simulink model "Top_Level"  (Simulink 7.5)
settings: Solver=ode45  StartTime=0.0  StopTime=inf  RelTol=1e-3
undefined symbols (not defined in the file): dfilt, DiscIntNeverNeededParam, fspecial, gray, Horn, imresize, Low, Rec, Schunck, SDTV
libraries: simulink x13, dspobslib x10, dspsigops x4, vipgeotforms x4, viptextngfix x4, vipsnks x3, dspmtrx3 x2, vipanalysis x2, vipconversions x1, dsparch4 x1, dspswit3 x1, vipsrcs x1
(part 1 of 2)
settings Model: Creator=roczit00  LastModifiedBy=Anonymos
settings DebuggingCC: AlgebraicLoopMsg=none  SolverPrmCheckMsg=none  UnconnectedInputMsg=none  UnconnectedOutputMsg=none  UnconnectedLineMsg=none  StrictBusMsg=Warning

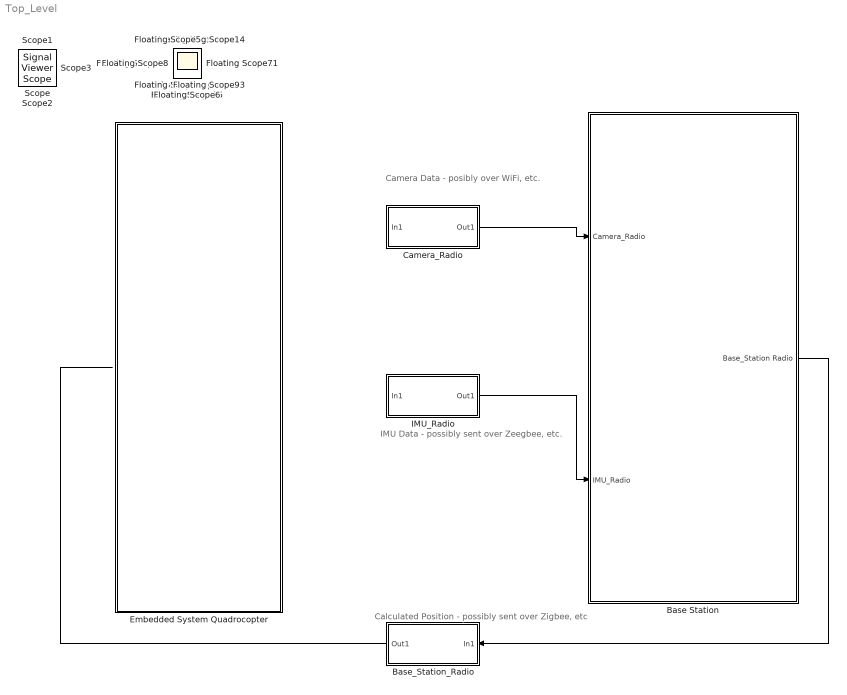
== system Top_Level ==
  note: IMU Data - possibly sent over Zeegbee, etc.
  note: Calculated Position - possibly sent over Zigbee, etc
  note: Camera Data - posibly over WiFi, etc.
  Base Station : Subsystem
  Base_Station_Radio : Subsystem
  Camera_Radio : Subsystem
  Embedded System Quadrocopter : Subsystem
  IMU_Radio : Subsystem
  Floating Scope{,1..15} (16 alike) : Scope
      Floating Scope settings: Floating=on  YMin=-40  YMax=90
      Floating Scope1 settings: Floating=on
      Floating Scope10 settings: Floating=on  SaveName=ScopeData12
      Floating Scope11 settings: Floating=on  SaveName=ScopeData13
      Floating Scope12 settings: Floating=on  YMin=-2500  YMax=27500  SaveName=ScopeData14
      Floating Scope13 settings: Floating=on  SaveName=ScopeData16
      Floating Scope14 settings: Floating=on  SaveName=ScopeData17
      Floating Scope15 settings: Floating=on  YMin=-2.5  YMax=27.5  SaveName=ScopeData18
      Floating Scope2 settings: Floating=on  YMin=-6000  YMax=2500  SaveName=ScopeData2
      Floating Scope3 settings: Floating=on  SaveName=ScopeData3
      Floating Scope4 settings: Floating=on  SaveName=ScopeData4
      Floating Scope5 settings: Floating=on  YMin=-0.7  YMax=0.8  SaveName=ScopeData5
      Floating Scope6 settings: Floating=on  YMin=-1  YMax=1  SaveName=ScopeData6
      Floating Scope7 settings: Floating=on  YMin=-15  YMax=10  SaveName=ScopeData7
      Floating Scope8 settings: Floating=on  YMax=45  SaveName=ScopeData10
      Floating Scope9 settings: Floating=on  YMin=-2  YMax=6.5  SaveName=ScopeData11
  Scope{,1..3} (4 alike) : SignalViewerScope  IOType=viewer  RefreshTime=0.035000
      Scope settings: YMin=-0.01  YMax=0.1
      Scope2 settings: SaveName=ScopeData2
      Scope3 settings: SaveName=ScopeData3
  wires:
  ? -> Camera_Radio/1(In1)
  Base Station/1(Base_Station Radio) -> Base_Station_Radio/1(In1)
  Base_Station_Radio/1(Out1) -> ?
  ? -> IMU_Radio/1(In1)
  IMU_Radio/1(Out1) -> Base Station/2(IMU_Radio)
  Camera_Radio/1(Out1) -> Base Station/1(Camera_Radio)

== system Top_Level/Base Station ==
  Camera_Radio : Inport
  IMU_Radio : Inport  Port=2
  Allow Image Processing : dspobslib/DSP Constant  SystemSampleTime=-1  Value=1  SampleMode=Discrete  discreteOutput=Sample-based  continuousOutput=Sample-based  sampTime=inf  framePeriod=2  dataType=boolean  isSigned=on  wordLen=16  udDataType=sfix(16)  fracBitsMode=Best precision  numFracBits=15  InterpretAs1D=-inf  Ts=-inf  FramebasedOutput=-inf
  Disable Image Processing : dspobslib/DSP Constant  SystemSampleTime=-1  Value=0  SampleMode=Discrete  discreteOutput=Sample-based  continuousOutput=Sample-based  sampTime=inf  framePeriod=2  dataType=boolean  isSigned=on  wordLen=16  udDataType=sfix(16)  fracBitsMode=Best precision  numFracBits=15  InterpretAs1D=-inf  Ts=-inf  FramebasedOutput=-inf
  Image Processing : Subsystem
  Selector1 : Selector  InputPortWidth=19  IndexOptions=Index vector (dialog)  Indices=[7 8 12]  OutputSizes=1
  Switch1 : simulink/Signal Routing/Manual Switch  SystemSampleTime=-1  sw=1  action=0  varsize=off
  Base_Station Radio : Outport
  wires:
  Camera_Radio/1 -> Selector1/1, Image Processing/1("x, y, vel_psi")
  Selector1/1 -> Base_Station Radio/1
  Allow Image Processing/1 -> Switch1/1
  Disable Image Processing/1 -> Switch1/2
  Switch1/1 -> Image Processing/Enable

== system Top_Level/Base_Station_Radio ==
  In1 : Inport
  Out1 : Outport
  wires:
  In1/1 -> Out1/1

== system Top_Level/Camera_Radio ==
  In1 : Inport
  Demux : Demux  Outputs=3
  Mux : Mux  Inputs=3
  Out1 : Outport
  wires:
  In1/1 -> Demux/1
  Demux/2 -> Mux/2
  Demux/3 -> Mux/3
  Demux/1 -> Mux/1
  Mux/1 -> Out1/1

== system Top_Level/Embedded System Quadrocopter ==

== system Top_Level/IMU_Radio ==
  In1 : Inport
  Out1 : Outport
  wires:
  In1/1 -> Out1/1

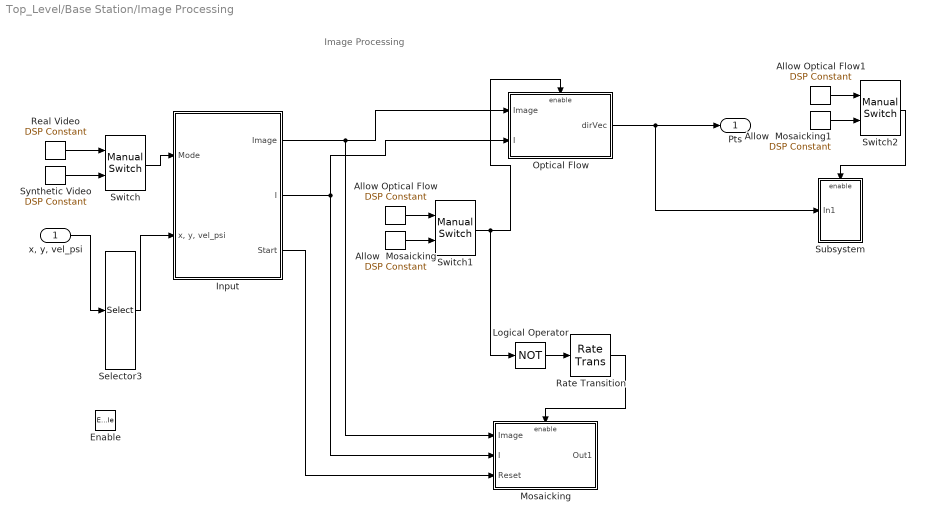
== system Top_Level/Base Station/Image Processing ==
  note: Image Processing
  "x, y, vel_psi" : Inport
  Enable : EnablePort  PropagateVarSize=During execution
  Allow  Mosaicking : dspobslib/DSP Constant  SystemSampleTime=-1  Value=0  SampleMode=Discrete  discreteOutput=Sample-based  continuousOutput=Sample-based  sampTime=inf  framePeriod=2  dataType=boolean  isSigned=on  wordLen=16  udDataType=sfix(16)  fracBitsMode=Best precision  numFracBits=15  InterpretAs1D=-inf  Ts=-inf  FramebasedOutput=-inf
  Allow  Mosaicking1 : dspobslib/DSP Constant  SystemSampleTime=-1  Value=0  SampleMode=Discrete  discreteOutput=Sample-based  continuousOutput=Sample-based  sampTime=inf  framePeriod=2  dataType=boolean  isSigned=on  wordLen=16  udDataType=sfix(16)  fracBitsMode=Best precision  numFracBits=15  InterpretAs1D=-inf  Ts=-inf  FramebasedOutput=-inf
  Allow Optical Flow : dspobslib/DSP Constant  SystemSampleTime=-1  Value=1  SampleMode=Discrete  discreteOutput=Sample-based  continuousOutput=Sample-based  sampTime=inf  framePeriod=2  dataType=boolean  isSigned=on  wordLen=16  udDataType=sfix(16)  fracBitsMode=Best precision  numFracBits=15  InterpretAs1D=-inf  Ts=-inf  FramebasedOutput=-inf
  Allow Optical Flow1 : dspobslib/DSP Constant  SystemSampleTime=-1  Value=1  SampleMode=Discrete  discreteOutput=Sample-based  continuousOutput=Sample-based  sampTime=inf  framePeriod=2  dataType=boolean  isSigned=on  wordLen=16  udDataType=sfix(16)  fracBitsMode=Best precision  numFracBits=15  InterpretAs1D=-inf  Ts=-inf  FramebasedOutput=-inf
  Input : Subsystem
  Logical Operator : Logic  Operator=NOT  AllPortsSameDT=off  OutDataTypeMode=boolean  OutDataTypeStr=boolean
  Mosaicking : Subsystem
  Optical Flow : Subsystem
  Rate Transition : RateTransition  OutPortSampleTimeOpt=Inherit
  Real Video : dspobslib/DSP Constant  SystemSampleTime=-1  Value=0  SampleMode=Discrete  discreteOutput=Sample-based  continuousOutput=Sample-based  sampTime=inf  framePeriod=2  dataType=boolean  isSigned=on  wordLen=16  udDataType=sfix(16)  fracBitsMode=Best precision  numFracBits=15  InterpretAs1D=-inf  Ts=-inf  FramebasedOutput=-inf
  Selector3 : Selector  InputPortWidth=19  IndexOptions=Index vector (dialog)  Indices=[1 2 6]  OutputSizes=1
  Subsystem : Subsystem
  Switch : simulink/Signal Routing/Manual Switch  SystemSampleTime=-1  sw=0  action=0  varsize=off
  Switch1 : simulink/Signal Routing/Manual Switch  SystemSampleTime=-1  sw=1  action=0  varsize=off
  Switch2 : simulink/Signal Routing/Manual Switch  SystemSampleTime=-1  sw=1  action=0  varsize=off
  Synthetic Video : dspobslib/DSP Constant  SystemSampleTime=-1  Value=1  SampleMode=Discrete  discreteOutput=Sample-based  continuousOutput=Sample-based  sampTime=inf  framePeriod=2  dataType=boolean  isSigned=on  wordLen=16  udDataType=sfix(16)  fracBitsMode=Best precision  numFracBits=15  InterpretAs1D=-inf  Ts=-inf  FramebasedOutput=-inf
  Pts : Outport  OutDataType=fixdt(1, 16)  OutScaling=2^0
  wires:
  Real Video/1 -> Switch/1
  Synthetic Video/1 -> Switch/2
  Switch/1 -> Input/1(Mode)
  "x, y, vel_psi"/1 -> Selector3/1
  Optical Flow/1(dirVec) -> Pts/1, Subsystem/1(In1)
  Input/1(Image) -> Mosaicking/1(Image), Optical Flow/1(Image)
  Input/2(I) -> Mosaicking/2(I), Optical Flow/2(I)
  Switch1/1 -> Optical Flow/Enable, Logical Operator/1
  Logical Operator/1 -> Rate Transition/1
  Rate Transition/1 -> Mosaicking/Enable
  Input/3(Start) -> Mosaicking/3(Reset)
  Allow Optical Flow/1 -> Switch1/1
  Allow  Mosaicking/1 -> Switch1/2
  Selector3/1 -> Input/2("x, y, vel_psi")
  Allow Optical Flow1/1 -> Switch2/1
  Allow  Mosaicking1/1 -> Switch2/2
  Switch2/1 -> Subsystem/Enable

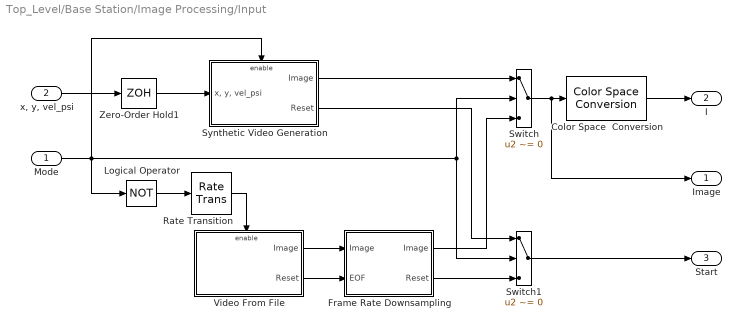
== system Top_Level/Base Station/Image Processing/Input ==
  Mode : Inport  OutDataType=sfix(16)  OutScaling=2^0
  "x, y, vel_psi" : Inport  Port=2  OutDataType=sfix(16)  OutScaling=2^0
  Color Space  Conversion : vipconversions/Color Space  Conversion  conversion=Obsolete  conversionActive=R'G'B' to intensity  wp_str=D65  rec=Rec. 601 (SDTV)  sys=1125/60/2:1  imagePorts=One multidimensional signal
  Frame Rate Downsampling : Subsystem  mask(Select Video Frames){frameRate=1}
      mask prompts: frameRate "N:"
      mask help: Downsample the video sequence by processing every Nth frame.
      mask init:
      | switch frameRate
      |     case 1,
      |         icon = sprintf('Select\nAll Frames');
      |     case 2,
      |         icon = sprintf('Select Every\n2nd Frame');
      |     case 3,
      |         icon = sprintf('Select Every\n3rd Frame');
      |     otherwise,
      |         icon = sprintf('Select Every\n%dth Frame',frameRate);
      | end
      mask Display: disp(icon);
  Logical Operator : Logic  Operator=NOT  AllPortsSameDT=off  OutDataTypeMode=boolean  OutDataTypeStr=boolean
  Rate Transition : RateTransition  OutPortSampleTimeOpt=Inherit
  Switch : Switch  Criteria=u2 ~= 0  OutDataType=sfix(16)  OutScaling=2^0
  Switch1 : Switch  Criteria=u2 ~= 0  OutDataType=sfix(16)  OutScaling=2^0
  Synthetic Video Generation : Subsystem  mask(Synthetic Video Generation){dimen=[288 352], origin=[509 765], velocity=[5 10], varVelocity=[8 5], varCorner=[10 10], rotation=1, varRotation=0.2}
      mask prompts: dimen "Size of the synthetic image:"; origin "Initial image center:"; varVelocity "Variance of velocity:"; varCorner "Variance of corner location:"; rotation "Rotation speed (in degrees):"; varRotation "Variation of rotation (in degrees):"
      mask help: Generates a synthetic video.
  Video From File : Subsystem
  Zero-Order Hold1 : ZeroOrderHold  SampleTime=0.01
  Image : Outport
  I : Outport  Port=2
  Start : Outport  Port=3
  wires:
  Switch1/1 -> Start/1
  Switch/1 -> Image/1, Color Space  Conversion/1
  Logical Operator/1 -> Rate Transition/1
  Rate Transition/1 -> Video From File/Enable
  Synthetic Video Generation/2(Reset) -> Switch1/1
  Synthetic Video Generation/1(Image) -> Switch/1
  Mode/1 -> Logical Operator/1, Switch1/2, Switch/2, Synthetic Video Generation/Enable
  Video From File/1(Image) -> Frame Rate Downsampling/1(Image)
  Video From File/2(Reset) -> Frame Rate Downsampling/2(EOF)
  Frame Rate Downsampling/1("Image ") -> Switch/3
  Frame Rate Downsampling/2(Reset) -> Switch1/3
  "x, y, vel_psi"/1 -> Zero-Order Hold1/1
  Zero-Order Hold1/1 -> Synthetic Video Generation/1("x, y, vel_psi")
  Color Space  Conversion/1 -> I/1

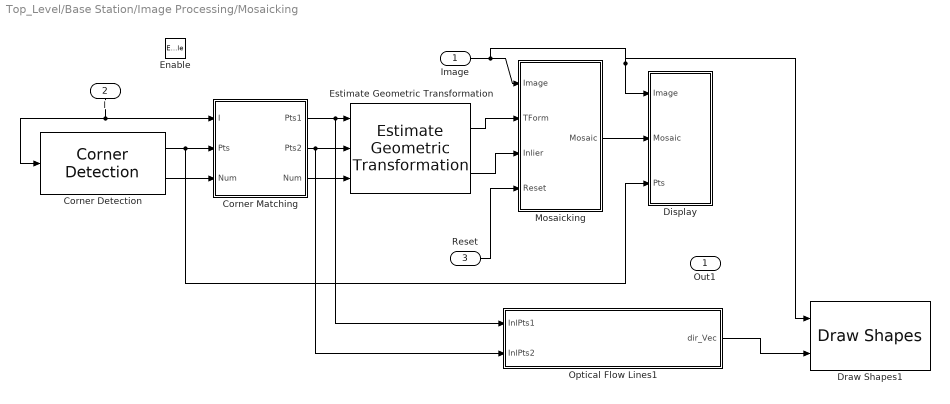
== system Top_Level/Base Station/Image Processing/Mosaicking ==
  Image : Inport
  I : Inport  Port=2
  Reset : Inport  Port=3
  Enable : EnablePort  PropagateVarSize=During execution
  Corner Detection : vipanalysis/Corner Detection  DialogController=vipDDGCreate  DialogControllerArgs=DataTag5  SystemSampleTime=-1  method=Local intensity comparison (Rosen & Drummond)  factor=0.04  filter=fspecial('gaussian', [1 5], 1.5)  thrInten=0.1  thrAngle=157.5  output=Corner location  outputInUse=Corner location  maxNum=75  thrMetric=0.001  neighborSize=[21 21]  isOutVarDim=on  accumMode=Binary point scaling  accumWordLength=32  accumFracLength=0  prodOutputMode=Binary point scaling  prodOutputWordLength=32  prodOutputFracLength=0  memoryMode=Binary point scaling  memoryWordLength=32  memoryFracLength=0  firstCoeffMode=Specify word length  firstCoeffWordLength=16  firstCoeffFracLength=16  roundingMode=Floor  overflowMode=off
  Corner Matching : Subsystem  mask(Corner Matching){winLen=9, maxNum=75, threshold=81}
      mask prompts: winLen "Block size used in corner matching:"; maxNum "Maximum number of points:"; threshold "Maximum feature difference for matching points:"
      mask help: Find out matching corners in the current and previous video frames.
  Display : Subsystem
  Draw Shapes1 : viptextngfix/Draw Shapes  DialogController=vipDDGCreate  DialogControllerArgs=DataTag13  shape=Lines  fill=off  fillClrSource=Specify via dialog  display=User-specified value  intensity=200  color=[255 255 0]  opacity=0.6  viewport=Entire image  antialiasing=off  inType=Obsolete  imagePorts=One multidimensional signal  prodOutputMode=Binary point scaling  prodOutputWordLength=32  prodOutputFracLength=14  memoryMode=Specify word length  memoryWordLength=16  memoryFracLength=15  roundingMode=Floor  overflowMode=off
  Estimate Geometric Transformation : vipgeotforms/Estimate Geometric Transformation  DialogController=vipDDGCreate  DialogControllerArgs=DataTag14  tformType=Projective  isRandomSampling=on  algMethod=Random Sample Consensus (RANSAC)  numMethod=Desired confidence  isStopSampling=on  percentStop=75  distanceAlg=1  distanceGeo=1.5  sampleNum=500  maxSampleNum=500  desiredConfidence=99  isRefineTForm=on  isOutputInlier=on  outDT4IntInput=Obsolete10a  outDT4IntInputActive=Single  isVarSizeAllowed=off  isReleaseMode=on
  Mosaicking : Subsystem  mask(Mosaicking){sizePano=[400 670], orginPano=[60 5]}
      mask prompts: sizePano "Size of the mosaic image:"; orginPano "Initial image placement (top-left image boundary):"
      mask help: Overlay video frames to create mosaic image.
  Optical Flow Lines1 : Stateflow chart  TreatAsAtomicUnit=on
  Out1 : Outport  OutDataType=fixdt(1, 16)  OutScaling=2^0
  wires:
  Corner Detection/1 -> Corner Matching/2(Pts), Display/3(Pts)
  Corner Detection/2 -> Corner Matching/3(Num)
  Mosaicking/1(Mosaic) -> Display/2(Mosaic)
  Corner Matching/1(Pts1) -> Estimate Geometric Transformation/1, Optical Flow Lines1/1(InlPts1)
  Corner Matching/2(Pts2) -> Estimate Geometric Transformation/2, Optical Flow Lines1/2(InlPts2)
  Corner Matching/3("Num ") -> Estimate Geometric Transformation/3
  Estimate Geometric Transformation/2 -> Mosaicking/3(Inlier)
  Estimate Geometric Transformation/1 -> Mosaicking/2(TForm)
  Image/1 -> Mosaicking/1(Image), Display/1(Image), Draw Shapes1/1
  I/1 -> Corner Detection/1, Corner Matching/1(I)
  Reset/1 -> Mosaicking/4(Reset)
  Optical Flow Lines1/1(dir_Vec) -> Draw Shapes1/2

== system Top_Level/Base Station/Image Processing/Optical Flow ==
  note: Optical Flow Movement Detection
  Image : Inport
  I : Inport  Port=2
  Enable : EnablePort  PropagateVarSize=During execution
  Allow draw lines : dspobslib/DSP Constant  SystemSampleTime=-1  Value=1  SampleMode=Discrete  discreteOutput=Sample-based  continuousOutput=Sample-based  sampTime=inf  framePeriod=2  dataType=boolean  isSigned=on  wordLen=16  udDataType=sfix(16)  fracBitsMode=Best precision  numFracBits=15  InterpretAs1D=-inf  Ts=-inf  FramebasedOutput=-inf
  Disable draw lines : dspobslib/DSP Constant  SystemSampleTime=-1  Value=0  SampleMode=Discrete  discreteOutput=Sample-based  continuousOutput=Sample-based  sampTime=inf  framePeriod=2  dataType=boolean  isSigned=on  wordLen=16  udDataType=sfix(16)  fracBitsMode=Best precision  numFracBits=15  InterpretAs1D=-inf  Ts=-inf  FramebasedOutput=-inf
  Optical Flow Lines1 : Subsystem  mask(Optical Flow Lines){scaleFactor=0.0008}
      mask prompts: scaleFactor "Motion vector gain:"
      mask help: Generates the coordinate points of optical flow lines.
      mask Help: Generates the coordinate points of optical flow lines. Look under its mask to see the implementation details.
  Optical Flow1 : vipanalysis/Optical Flow  DialogController=vipDDGCreate  DialogControllerArgs=DataTag17  SystemSampleTime=-1  method=Horn-Schunck  gradMethod=Derivative of Gaussian  which2img=Current frame and N-th frame back  N=1  outVelForm=Horizontal and vertical components in complex form  lambda=0.01  stop_criteria=When maximum number of iterations is reached  maxAllowAbsDiff=eps  maxIter=10  numInports=3  sigmaS=1.5  sigmaW=1  eigTh=0.0039  discardNormalFlow=off  outputCurrentImage=on  prodOutputMode=Binary point scaling  prodOutputWordLength=32  prodOutputFracLength=20  outputMode=Binary point scaling  outputWordLength=32  outputFracLength=20  roundingMode=Nearest  overflowMode=on
  Subsystem : Subsystem
  Switch2 : simulink/Signal Routing/Manual Switch  SystemSampleTime=-1  sw=1  action=0  varsize=off
  dirVec : Outport  OutDataType=fixdt(1, 16)  OutScaling=2^0
  wires:
  Optical Flow1/1 -> Optical Flow Lines1/1(vel.Values)
  Optical Flow Lines1/1(vel.Lines) -> Subsystem/2(In2)
  Image/1 -> Subsystem/1(In1)
  I/1 -> Optical Flow1/1
  Optical Flow Lines1/2(dirVec) -> dirVec/1
  Allow draw lines/1 -> Switch2/1
  Disable draw lines/1 -> Switch2/2
  Switch2/1 -> Subsystem/Enable

== system Top_Level/Base Station/Image Processing/Subsystem ==
  In1 : Inport
  Enable : EnablePort  PropagateVarSize=During execution
  Demux : Demux  Outputs=2
  Discrete-Time Integrator : DiscreteIntegrator  SampleTime=-1  OutDataType=fixdt(1, 16)  OutScaling=2^0  ICPrevOutput=DiscIntNeverNeededParam  ICPrevScaledInput=DiscIntNeverNeededParam
  Gain1 : Gain  Gain=-1  ParameterDataType=fixdt(1, 16)  ParameterScaling=2^0  OutDataType=fixdt(1, 16)  OutScaling=2^0
  XY Pos. Est : simulink/Sinks/XY Graph  SystemSampleTime=-1  xmin=-10  xmax=10  ymin=-10  ymax=10  st=-1
  wires:
  Discrete-Time Integrator/1 -> Demux/1
  Demux/1 -> XY Pos. Est/1
  Demux/2 -> Gain1/1
  Gain1/1 -> XY Pos. Est/2
  In1/1 -> Discrete-Time Integrator/1

== system Top_Level/Base Station/Image Processing/Input/Frame Rate Downsampling ==
  Image : Inport  OutDataType=sfix(16)  OutScaling=2^0
  EOF : Inport  Port=2  OutDataType=sfix(16)  OutScaling=2^0
  Compare To Zero : simulink/Logic and Bit Operations/Compare To Zero  SystemSampleTime=-1  relop=>  LogicOutDataTypeMode=boolean  ZeroCross=off
  Data Type Conversion : DataTypeConversion  OutDataTypeMode=single  OutDataType=sfix(16)  OutScaling=2^0  OutDataTypeStr=single
  Digital Filter : dsparch4/Digital Filter  DialogController=dspdialog.DigitalFilter  DialogControllerArgs=DataTag0  TypePopup=FIR (all zeros)  IIRFiltStruct=Direct form II transposed  AllPoleFiltStruct=Direct form  FIRFiltStruct=Direct form  CoeffSource=Specify via dialog  NumCoeffs=ones(1, frameRate)  DenCoeffs=[1 0.1]  BiQuadCoeffs=[1 0.3 0.4 1 0.1 0.2]  LatticeCoeffs=[0.2 0.4]  denIgnore=on  FiltPerSampPopup=One filter per frame  IC=0  ICnum=0  ICden=0  roundingMode=Floor  overflowMode=off  ScaleValues=1  scaleValueFracLength=14  stageInFracLength=15  stageOutFracLength=15  FilterSource=Specify via dialog  dfiltObjectName=dfilt.dffir([1 2 1])
  Downsample : dspsigops/Downsample  N=frameRate  phase=0  ic=0  smode=Allow multirate  fmode=Maintain input frame size
  Downsample3 : dspsigops/Downsample  N=frameRate  phase=0  ic=0  smode=Allow multirate  fmode=Maintain input frame size
  Unit Delay : UnitDelay  X0=1  SampleTime=-1
  "Image " : Outport  OutDataType=sfix(16)  OutScaling=2^0
  Reset : Outport  Port=2
  wires:
  Digital Filter/1 -> Compare To Zero/1
  Data Type Conversion/1 -> Digital Filter/1
  Compare To Zero/1 -> Unit Delay/1
  Downsample3/1 -> Reset/1
  EOF/1 -> Data Type Conversion/1
  Unit Delay/1 -> Downsample3/1
  Image/1 -> Downsample/1
  Downsample/1 -> "Image "/1

== system Top_Level/Base Station/Image Processing/Input/Synthetic Video Generation ==
  "x, y, vel_psi" : Inport  OutDataType=sfix(16)  OutScaling=2^0
  Enable : EnablePort  PropagateVarSize=During execution
  N-Sample Enable : dspswit3/N-Sample Enable  N=1  ActiveLevel=Low (0)  reset=off  TriggerType=Rising edge  Ts=-1  DataType=Logical
  Read Image : Subsystem
      settings: AttributesFormatString=Load image only at the beginning of simulation
  Synthesize Video : Subsystem  mask{dimen=dimen, origin=origin, velocity=velocity, varVelocity=varVelocity, varCorner=varCorner, rotation=rotation, varRotation=varRotation}
      mask prompts: dimen "Size of the synthetic image:"; origin "Initial image center:"; varVelocity "Variance of velocity:"; varCorner "Variance of corner location:"; rotation "Rotation speed:"; varRotation "Variation of rotation:"
  Image : Outport
  Reset : Outport  Port=2  InitialOutput=1
  wires:
  Read Image/2(Size) -> Synthesize Video/2(Size)
  Read Image/1(Image) -> Synthesize Video/1("Image ")
  N-Sample Enable/1 -> Read Image/Enable
  Synthesize Video/2(Reset) -> Reset/1
  Synthesize Video/1(Image) -> Image/1
  "x, y, vel_psi"/1 -> Synthesize Video/3("x, y, vel_psi")

== system Top_Level/Base Station/Image Processing/Input/Video From File ==
  Enable : EnablePort  PropagateVarSize=During execution
  From Multimedia File : dspsrcs4/From Multimedia File  DialogController=dspDDGCreate  DialogControllerArgs=DataTag4  inputFilename=D:\_HSE\_ARBEIT\eclipse-cpp-galileo-SR1-win32\Workspace2\MASTER_THESIS_PRJ\scratch\Ground_Videos\grey_amorphic_flow_tiles_variable_light.avi  loop=on  numPlays=inf  outputStreams=Video only  videoDataType=single  audioDataType=int16  inheritSampleTime=on  userDefinedSampleTime=1/30  noAudioOutput=off  isIntensityVideo=off  fourcc=RGB  colorVideoFormat=One multidimensional signal  outputEOF=on  dataOrg=Column-major  audioFrameSize=1024  computeAudioFrameSize=off
  Image : Outport
  Reset : Outport  Port=2
  wires:
  From Multimedia File/1 -> Image/1
  From Multimedia File/2 -> Reset/1

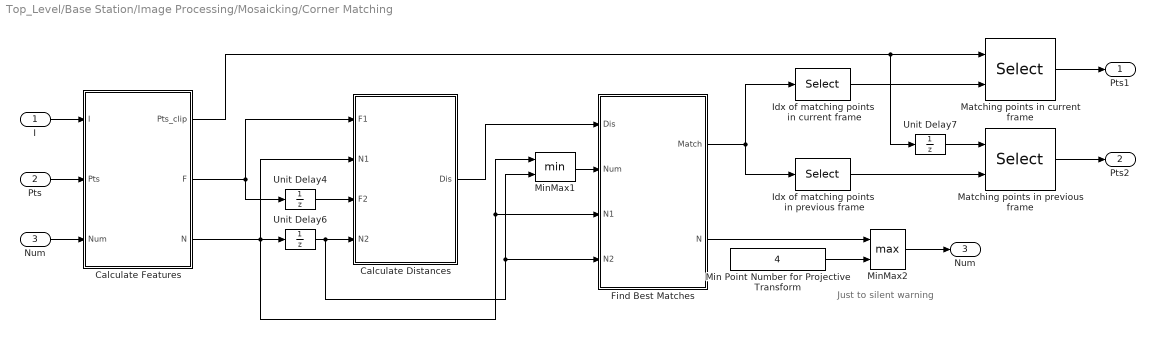
== system Top_Level/Base Station/Image Processing/Mosaicking/Corner Matching ==
  note: Just to
      | silent warning
  I : Inport  OutDataType=sfix(16)  OutScaling=2^0
  Pts : Inport  Port=2  OutDataType=sfix(16)  OutScaling=2^0
  Num : Inport  Port=3  OutDataType=sfix(16)  OutScaling=2^0
  Calculate Distances : Subsystem  TreatAsAtomicUnit=on  mask{maxNum=maxNum}
      mask prompts: maxNum "Maximum data number:"
      settings: AttributesFormatString=between features.
  Calculate Features : Subsystem  TreatAsAtomicUnit=on  mask{winLen=winLen, maxNum=maxNum}
      mask prompts: winLen "Neighborhood size:"; maxNum "Maximum number of features:"
  Find Best Matches : Subsystem  TreatAsAtomicUnit=on  mask{maxNum=maxNum, threshold=threshold}
      mask prompts: maxNum "Maximum data number:"
      settings: AttributesFormatString=between the features\nin the current and previous frames
  Idx of matching points  in current frame : Selector  NumberOfDimensions=2  IndexMode=Zero-based  InputPortWidth=2  IndexOptions=Index vector (dialog),Select all  Indices=0,1  OutputSizes=1,1
  Idx of matching points  in previous frame : Selector  NumberOfDimensions=2  IndexMode=Zero-based  InputPortWidth=2  IndexOptions=Index vector (dialog),Select all  Indices=1,1  OutputSizes=1,1
  Matching points in current frame : Selector  NumberOfDimensions=2  IndexMode=Zero-based  InputPortWidth=2  IndexOptions=Select all,Index vector (port)  Indices=0,1  OutputSizes=1,1
  Matching points in previous frame : Selector  NumberOfDimensions=2  IndexMode=Zero-based  InputPortWidth=2  IndexOptions=Select all,Index vector (port)  Indices=0,1  OutputSizes=1,1
  Min Point Number for Projective Transform : Constant  Value=4  OutDataType=sfix(16)  OutScaling=2^0  OutDataTypeStr=Inherit: Inherit via back propagation
  MinMax1 : MinMax  Inputs=2  OutDataType=sfix(16)  OutScaling=2^0
  MinMax2 : MinMax  Function=max  Inputs=2  OutDataType=sfix(16)  OutScaling=2^0  OutDataTypeStr=Inherit: Inherit via back propagation
  Unit Delay4 : UnitDelay  SampleTime=-1
  Unit Delay6 : UnitDelay  SampleTime=-1
  Unit Delay7 : UnitDelay  SampleTime=-1
  Pts1 : Outport  OutDataType=sfix(16)  OutScaling=2^0
  Pts2 : Outport  Port=2  OutDataType=sfix(16)  OutScaling=2^0
  "Num " : Outport  Port=3  OutDataType=sfix(16)  OutScaling=2^0
  wires:
  Calculate Features/2(F) -> Calculate Distances/1(F1), Unit Delay4/1
  Calculate Features/3(N) -> Calculate Distances/2(N1), Unit Delay6/1, MinMax1/1, Find Best Matches/3(N1)
  Calculate Features/1(Pts_clip) -> Unit Delay7/1, Matching points in current frame/1
  Num/1 -> Calculate Features/3(Num)
  Unit Delay6/1 -> Calculate Distances/4(N2), MinMax1/2, Find Best Matches/4(N2)
  Unit Delay4/1 -> Calculate Distances/3(F2)
  Matching points in previous frame/1 -> Pts2/1
  Matching points in current frame/1 -> Pts1/1
  Unit Delay7/1 -> Matching points in previous frame/1
  Idx of matching points  in current frame/1 -> Matching points in current frame/2
  Idx of matching points  in previous frame/1 -> Matching points in previous frame/2
  Find Best Matches/1(Match) -> Idx of matching points  in previous frame/1, Idx of matching points  in current frame/1
  Calculate Distances/1(Dis) -> Find Best Matches/1(Dis)
  I/1 -> Calculate Features/1(I)
  Pts/1 -> Calculate Features/2(Pts)
  Min Point Number for Projective Transform/1 -> MinMax2/2
  Find Best Matches/2(N) -> MinMax2/1
  MinMax2/1 -> "Num "/1
  MinMax1/1 -> Find Best Matches/2(Num)

== system Top_Level/Base Station/Image Processing/Mosaicking/Display ==
  Image : Inport  OutDataType=sfix(16)  OutScaling=2^0
  Mosaic : Inport  Port=2  OutDataType=sfix(16)  OutScaling=2^0
  Pts : Inport  Port=3  OutDataType=sfix(16)  OutScaling=2^0
  Corners : vipsnks/Video Viewer  DialogControllerArgs=DataTag9  inputType=Obsolete7b  imagePorts=One multidimensional signal  useColorMap=off  colormapValue=gray(256)  specRange=off  minInputVal=0  maxInputVal=255  FigPos=[1 766 1276 659]  AxisZoom=on  trueSizedOnce=on  OpenAtMdlStart=on
  Draw Corners : viptextngfix/Draw Markers  DialogController=vipDDGCreate  DialogControllerArgs=DataTag10  shape=Circle  size=3  fill=off  fillClrSource=Specify via dialog  display=User-specified value  intensity=155  color=[1 0 0]  opacity=1  viewport=Entire image  antialiasing=off  inType=Obsolete  imagePorts=One multidimensional signal  prodOutputMode=Binary point scaling  prodOutputWordLength=32  prodOutputFracLength=14  memoryMode=Specify word length  memoryWordLength=16  memoryFracLength=15  roundingMode=Floor  overflowMode=off
  "Mosaic " : vipsnks/Video Viewer  DialogControllerArgs=DataTag12  inputType=Obsolete7b  imagePorts=One multidimensional signal  useColorMap=off  colormapValue=gray(256)  specRange=off  minInputVal=0  maxInputVal=255  FigPos=[12 653 673 423]  AxisZoom=on  trueSizedOnce=on  OpenAtMdlStart=on
  wires:
  Mosaic/1 -> "Mosaic "/1
  Image/1 -> Draw Corners/1
  Draw Corners/1 -> Corners/1
  Pts/1 -> Draw Corners/2

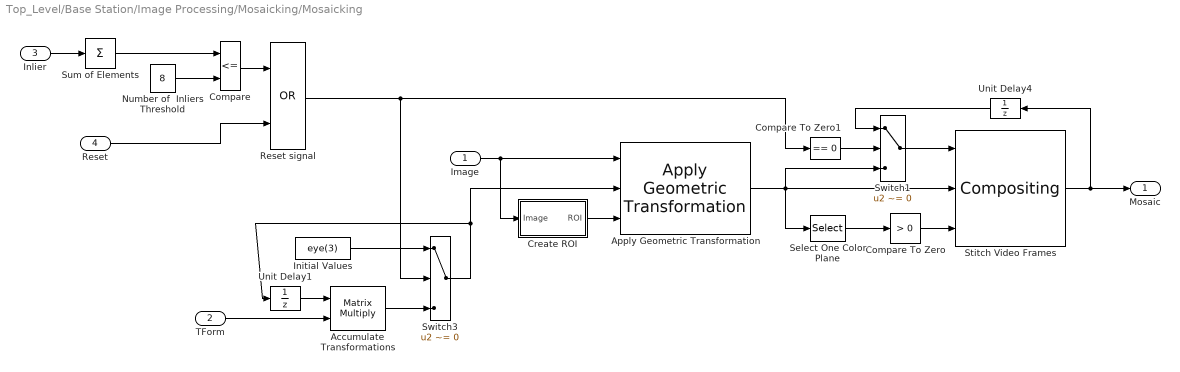
== system Top_Level/Base Station/Image Processing/Mosaicking/Mosaicking ==
  Image : Inport  OutDataType=sfix(16)  OutScaling=2^0
  TForm : Inport  Port=2  OutDataType=sfix(16)  OutScaling=2^0
  Inlier : Inport  Port=3  OutDataType=sfix(16)  OutScaling=2^0
  Reset : Inport  Port=4  OutDataType=sfix(16)  OutScaling=2^0
  Accumulate Transformations : Product  Multiplication=Matrix(*)  OutDataType=sfix(16)  OutScaling=2^0  RndMeth=Zero  InputSameDT=on
  Apply Geometric Transformation : vipgeotforms/Apply Geometric Transformation  DialogController=vipDDGCreate  DialogControllerArgs=DataTag15  tformSource=Input port  tformValue=[1 0 0; 0 1 0; 0 0 1]  approxProjectiveFlag=off  errorTolerance=1.0  roiMethod=Rectangle ROI  roiSource=Input port  roiBBox=[0 0 128 256]  roiVertice=[0 0 10 12 20 22]  inputClipFlag=off  interpolationMethod=Bilinear  fillValue=0  viewPortMethod=Specify via dialog  outputSize=sizePano  outputLoc=-orginPano  outputClipFlag=off
  Compare : RelationalOperator  Operator=<=  LogicOutDataTypeMode=boolean  OutDataTypeStr=boolean  ZeroCross=off  InputSameDT=on
  Compare To Zero : simulink/Logic and Bit Operations/Compare To Zero  SystemSampleTime=-1  relop=>  LogicOutDataTypeMode=boolean  ZeroCross=off
  Compare To Zero1 : simulink/Logic and Bit Operations/Compare To Zero  SystemSampleTime=-1  relop===  LogicOutDataTypeMode=boolean  ZeroCross=off
  Create ROI : Subsystem
  Initial Values : Constant  Value=eye(3)  OutDataType=sfix(16)  OutScaling=2^0  OutDataTypeStr=Inherit: Inherit via back propagation  SampleTime=-1
  Number of  Inliers Threshold : Constant  Value=8  OutDataType=sfix(16)  OutScaling=1  OutDataTypeStr=Inherit: Inherit via back propagation  SampleTime=-1
  Reset signal : Logic  Operator=OR  AllPortsSameDT=off  OutDataTypeMode=boolean  OutDataTypeStr=boolean
      settings: AttributesFormatString=Restart mosaicking when the video started\nor when no enough inliers were found.
  Select One Color Plane : Selector  NumberOfDimensions=3  InputPortWidth=3  IndexOptions=Select all,Select all,Index vector (dialog)  Indices=40,10,1  OutputSizes=240,320,1
  Stitch Video Frames : viptextngfix/Compositing  DialogController=vipDDGCreate  DialogControllerArgs=DataTag16  operation=Binary mask  bFacSrc=Specify via dialog  mFacSrc=Input port  bFactor=0.2  mFactor=1  source=Specify via dialog  coordinates=[0 0]  prodOutputMode=Binary point scaling  prodOutputWordLength=32  prodOutputFracLength=10  roundingMode=Floor  overflowMode=off
  Sum of Elements : Sum  Inputs=+  OutDataType=sfix(16)  OutScaling=2^-10
  Switch1 : Switch  Criteria=u2 ~= 0  OutDataType=sfix(16)  OutScaling=2^0  ZeroCross=off  InputSameDT=on
  Switch3 : Switch  Criteria=u2 ~= 0  OutDataType=sfix(16)  OutScaling=2^0  ZeroCross=off  InputSameDT=on
  Unit Delay1 : UnitDelay  SampleTime=-1
  Unit Delay4 : UnitDelay  SampleTime=-1
  Mosaic : Outport  OutDataType=sfix(16)  OutScaling=2^0
  wires:
  Reset/1 -> Reset signal/2
  Compare/1 -> Reset signal/1
  Unit Delay4/1 -> Switch1/1
  Inlier/1 -> Sum of Elements/1
  Number of  Inliers Threshold/1 -> Compare/2
  Sum of Elements/1 -> Compare/1
  Switch3/1 -> Unit Delay1/1, Apply Geometric Transformation/2
  Reset signal/1 -> Switch3/2, Compare To Zero1/1
  TForm/1 -> Accumulate Transformations/2
  Accumulate Transformations/1 -> Switch3/3
  Unit Delay1/1 -> Accumulate Transformations/1
  Initial Values/1 -> Switch3/1
  Select One Color Plane/1 -> Compare To Zero/1
  Apply Geometric Transformation/1 -> Stitch Video Frames/2, Select One Color Plane/1, Switch1/3
  Stitch Video Frames/1 -> Unit Delay4/1, Mosaic/1
  Switch1/1 -> Stitch Video Frames/1
  Compare To Zero/1 -> Stitch Video Frames/3
  Compare To Zero1/1 -> Switch1/2
  Image/1 -> Apply Geometric Transformation/1, Create ROI/1(Image)
  Create ROI/1(ROI) -> Apply Geometric Transformation/3

== system Top_Level/Base Station/Image Processing/Optical Flow/Optical Flow Lines1 ==
  vel.Values : Inport  OutDataType=sfix(16)  OutScaling=2^0
  Optical Flow Lines1 : Stateflow chart  TreatAsAtomicUnit=on
  vel.Lines : Outport  OutDataType=sfix(16)  OutScaling=2^0
  dirVec : Outport  Port=2  OutDataType=sfix(16)  OutScaling=2^0
  wires:
  Optical Flow Lines1/1(vel_Lines) -> vel.Lines/1
  vel.Values/1 -> Optical Flow Lines1/1(vel_Values)
  Optical Flow Lines1/2(dir_Vec) -> dirVec/1

== system Top_Level/Base Station/Image Processing/Optical Flow/Subsystem ==
  In1 : Inport
  In2 : Inport  Port=2
  Enable : EnablePort  PropagateVarSize=During execution
  Draw Shapes1 : viptextngfix/Draw Shapes  DialogController=vipDDGCreate  DialogControllerArgs=DataTag18  shape=Lines  fill=off  fillClrSource=Specify via dialog  display=User-specified value  intensity=200  color=[255 255 0]  opacity=0.6  viewport=Entire image  antialiasing=off  inType=Obsolete  imagePorts=One multidimensional signal  prodOutputMode=Binary point scaling  prodOutputWordLength=32  prodOutputFracLength=14  memoryMode=Specify word length  memoryWordLength=16  memoryFracLength=15  roundingMode=Floor  overflowMode=off
  To Video Display : vipsnks/To Video Display  DialogControllerArgs=DataTag19  inputType=Obsolete  imagePorts=One multidimensional signal  OutputDevice=On-screen video monitor  fullScreen=off  videoWindowX=111  videoWindowY=18  saveWindowSize=off  videoWindowWidth=352  videoWindowHeight=288  dataOrg=Column-major  openAtMdlStart=on  isWindowOpen=on
  wires:
  Draw Shapes1/1 -> To Video Display/1
  In1/1 -> Draw Shapes1/1
  In2/1 -> Draw Shapes1/2

== system Top_Level/Base Station/Image Processing/Input/Synthetic Video Generation/Read Image ==
  Enable : EnablePort  PropagateVarSize=During execution
  Image From Workspace : vipsrcs/Image From Workspace  Tag=vipblks_nd  SystemSampleTime=-1  ImageValue=imresize(imread('concordaerial.png'), 0.5)  Ts=inf  imagePorts=One multidimensional signal  ImageDataType=single  Signed=on  WordLength=16  sdImageDataType=sfix(16)  FractionLengthMode=User-defined  FractionLength=15  OutPortLabels=R|G|B
  Probe : Probe  ProbeWidth=off  ProbeSampleTime=off  ProbeComplexSignal=off  ProbeSignalDimensions=on  ProbeDimensionsDataType=single
  Image : Outport  InitialOutput=0
  Size : Outport  Port=2
  wires:
  Image From Workspace/1 -> Probe/1, Image/1
  Probe/1 -> Size/1

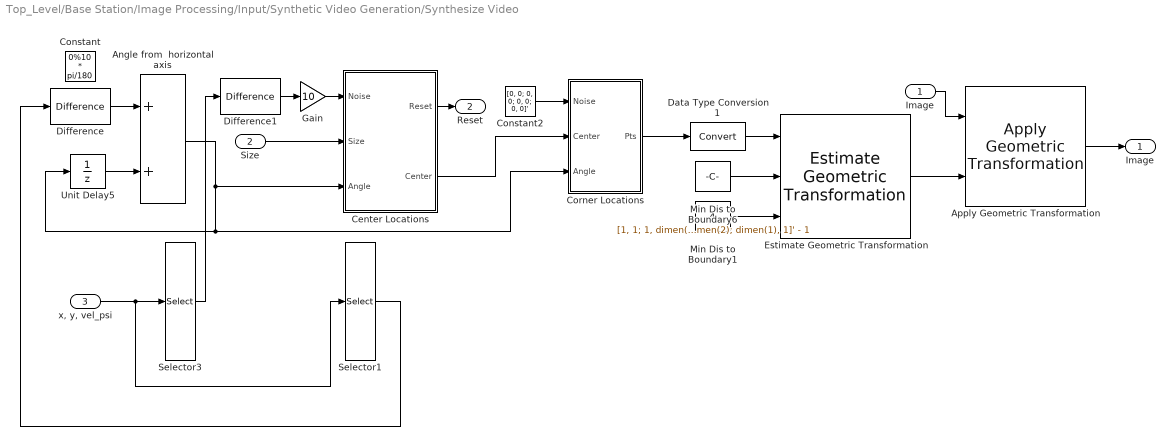
== system Top_Level/Base Station/Image Processing/Input/Synthetic Video Generation/Synthesize Video ==
  "Image " : Inport  OutDataType=sfix(16)  OutScaling=2^0
  Size : Inport  Port=2  OutDataType=sfix(16)  OutScaling=2^0
  "x, y, vel_psi" : Inport  Port=3  OutDataType=sfix(16)  OutScaling=2^0
  Angle from  horizontal axis : Sum  OutDataType=sfix(16)  OutScaling=2^-10
  Apply Geometric Transformation : vipgeotforms/Apply Geometric Transformation  DialogController=vipDDGCreate  DialogControllerArgs=DataTag1  tformSource=Input port  tformValue=[1 0 0; 0 1 0; 0 0 1]  approxProjectiveFlag=off  errorTolerance=1.0  roiMethod=Whole input image  roiSource=Specify via dialog  roiBBox=[0 0 128 256]  roiVertice=[0 0 10 12 20 22]  inputClipFlag=off  interpolationMethod=Bilinear  fillValue=0  viewPortMethod=Specify via dialog  outputSize=dimen  outputLoc=[0 0]  outputClipFlag=off
  Center Locations : Subsystem
  Constant : Constant  Value=0%10 * pi/180  OutDataType=fixdt(1, 16)  OutScaling=2^0
  Constant2 : Constant  Value=[0, 0; 0, 0; 0, 0; 0, 0]'  OutDataType=fixdt(1, 16)  OutScaling=2^0
  Corner Locations : Subsystem
  Data Type Conversion1 : DataTypeConversion  OutDataType=sfix(16)  OutScaling=2^0
  Difference : simulink/Discrete/Difference  SystemSampleTime=-1  ICPrevInput=0.0  OutMin=[]  OutMax=[]  OutDataType=fixdt(1, 16)  OutScaling=2^-10  DoSatur=off
  Difference1 : simulink/Discrete/Difference  SystemSampleTime=-1  ICPrevInput=0.0  OutMin=[]  OutMax=[]  OutDataType=fixdt(1, 16)  OutScaling=2^-10  DoSatur=off
  Estimate Geometric Transformation : vipgeotforms/Estimate Geometric Transformation  DialogController=vipDDGCreate  DialogControllerArgs=DataTag3  tformType=Projective  isRandomSampling=off  algMethod=Random Sample Consensus (RANSAC)  numMethod=Specified value  isStopSampling=off  percentStop=75  distanceAlg=1.5  distanceGeo=1.5  sampleNum=100  maxSampleNum=200  desiredConfidence=99  isRefineTForm=off  isOutputInlier=off  outDT4IntInput=Obsolete10a  outDT4IntInputActive=Single  isVarSizeAllowed=off  isReleaseMode=on
  Gain : Gain  Gain=10  ParameterDataType=fixdt(1, 16)  ParameterScaling=2^0  OutDataType=fixdt(1, 16)  OutScaling=2^0
  Min Dis to Boundary1 : Constant  Value=4  OutDataType=sfix(16)  OutScaling=2^0  OutDataTypeStr=Inherit: Inherit via back propagation
  Min Dis to Boundary6 : Constant  Value=[1, 1; 1, dimen(2); dimen(1), dimen(2); dimen(1), 1]' - 1  OutDataType=sfix(16)  OutScaling=2^0  OutDataTypeStr=Inherit: Inherit via back propagation
  Selector1 : Selector  InputPortWidth=3  IndexOptions=Index vector (dialog)  Indices=[3]  OutputSizes=1
  Selector3 : Selector  InputPortWidth=3  IndexOptions=Index vector (dialog)  Indices=[1 2]  OutputSizes=1
  Unit Delay5 : UnitDelay  X0=-pi/12  SampleTime=-1
  Image : Outport  OutDataType=sfix(16)  OutScaling=2^0
  Reset : Outport  Port=2  OutDataType=sfix(16)  OutScaling=2^0
  wires:
  Constant2/1 -> Corner Locations/1(Noise)
  Angle from  horizontal axis/1 -> Center Locations/3(Angle), Corner Locations/3(Angle), Unit Delay5/1
  Center Locations/1(Reset) -> Reset/1
  Size/1 -> Center Locations/2(Size)
  Min Dis to Boundary6/1 -> Estimate Geometric Transformation/2
  Min Dis to Boundary1/1 -> Estimate Geometric Transformation/3
  Data Type Conversion1/1 -> Estimate Geometric Transformation/1
  Estimate Geometric Transformation/1 -> Apply Geometric Transformation/2
  Corner Locations/1(Pts) -> Data Type Conversion1/1
  "x, y, vel_psi"/1 -> Selector3/1, Selector1/1
  Center Locations/2(Center) -> Corner Locations/2(Center)
  "Image "/1 -> Apply Geometric Transformation/1
  Apply Geometric Transformation/1 -> Image/1
  Unit Delay5/1 -> Angle from  horizontal axis/2
  Selector1/1 -> Difference/1
  Selector3/1 -> Difference1/1
  Difference/1 -> Angle from  horizontal axis/1
  Difference1/1 -> Gain/1
  Gain/1 -> Center Locations/1(Noise)

== system Top_Level/Base Station/Image Processing/Mosaicking/Corner Matching/Calculate Distances ==
  F1 : Inport  OutDataType=sfix(16)  OutScaling=2^0
  N1 : Inport  Port=2  OutDataType=sfix(16)  OutScaling=2^0
  F2 : Inport  Port=3  OutDataType=sfix(16)  OutScaling=2^0
  N2 : Inport  Port=4  OutDataType=sfix(16)  OutScaling=2^0
  For Iterator Subsystem : Subsystem  TreatAsAtomicUnit=on
  Initial Values1 : Constant  Value=maxNum  OutDataType=sfix(16)  OutScaling=2^0  OutDataTypeStr=Inherit: Inherit via back propagation  SampleTime=-1
  Initial Values2 : Constant  Value=maxNum  OutDataType=sfix(16)  OutScaling=2^0  OutDataTypeStr=Inherit: Inherit via back propagation  SampleTime=-1
  MinMax1 : MinMax  Inputs=2  OutDataType=sfix(16)  OutScaling=2^0
  MinMax2 : MinMax  Inputs=2  OutDataType=sfix(16)  OutScaling=2^0
  Dis : Outport  OutDataType=sfix(16)  OutScaling=2^0
  wires:
  MinMax2/1 -> For Iterator Subsystem/4(N2)
  F2/1 -> For Iterator Subsystem/3(F2)
  MinMax1/1 -> For Iterator Subsystem/2(N1)
  F1/1 -> For Iterator Subsystem/1(F1)
  For Iterator Subsystem/1(Dis) -> Dis/1
  N2/1 -> MinMax2/2
  Initial Values2/1 -> MinMax2/1
  N1/1 -> MinMax1/2
  Initial Values1/1 -> MinMax1/1

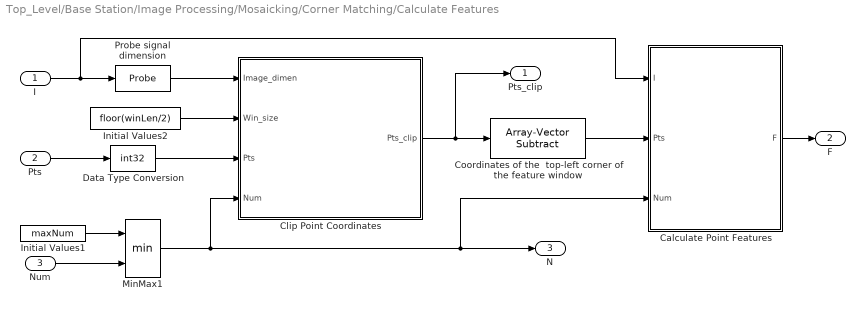
== system Top_Level/Base Station/Image Processing/Mosaicking/Corner Matching/Calculate Features ==
  I : Inport  OutDataType=sfix(16)  OutScaling=2^0
  Pts : Inport  Port=2  OutDataType=sfix(16)  OutScaling=2^0
  Num : Inport  Port=3  OutDataType=sfix(16)  OutScaling=2^0
  Calculate Point Features : Subsystem
  Clip Point Coordinates : Subsystem
  Coordinates of the  top-left corner of the feature window : dspmtrx3/Array-Vector Subtract  DialogController=dspDDGCreate  DialogControllerArgs=DataTag6  Dimension=1  V_Source=Dialog parameter  V_VectFromMask=floor([winLen; winLen] / 2)  firstCoeffDataTypeStr=Inherit: Same word length as input  firstCoeffLastDataTypeStr=Inherit: Same word length as input  firstCoeffMin=[]  firstCoeffMax=[]  outputMin=[]  outputMax=[]  roundingMode=Floor  overflowMode=off
  Data Type Conversion : DataTypeConversion  OutDataTypeMode=int32  OutDataType=sfix(16)  OutScaling=2^0  OutDataTypeStr=int32
  Initial Values1 : Constant  Value=maxNum  OutDataType=sfix(16)  OutScaling=2^0  OutDataTypeStr=Inherit: Inherit via back propagation  SampleTime=-1
  Initial Values2 : Constant  Value=floor(winLen/2)  OutDataType=sfix(16)  OutScaling=2^0  OutDataTypeStr=Inherit: Inherit via back propagation  SampleTime=-1
  MinMax1 : MinMax  Inputs=2  OutDataType=sfix(16)  OutScaling=2^0
  Probe signal dimension : Probe  ProbeWidth=off  ProbeSampleTime=off  ProbeComplexSignal=off  ProbeSignalDimensions=on  ProbeDimensionsDataType=int32
  Pts_clip : Outport  OutDataType=sfix(16)  OutScaling=2^0
  F : Outport  Port=2  OutDataType=sfix(16)  OutScaling=2^0
  N : Outport  Port=3  OutDataType=sfix(16)  OutScaling=2^0
  wires:
  Data Type Conversion/1 -> Clip Point Coordinates/3(Pts)
  MinMax1/1 -> N/1, Calculate Point Features/3(Num), Clip Point Coordinates/4(Num)
  Coordinates of the  top-left corner of the feature window/1 -> Calculate Point Features/2(Pts)
  Clip Point Coordinates/1(Pts_clip) -> Coordinates of the  top-left corner of the feature window/1, Pts_clip/1
  Pts/1 -> Data Type Conversion/1
  Initial Values2/1 -> Clip Point Coordinates/2(Win_size)
  Probe signal dimension/1 -> Clip Point Coordinates/1(Image_dimen)
  I/1 -> Calculate Point Features/1(I), Probe signal dimension/1
  Initial Values1/1 -> MinMax1/1
  Num/1 -> MinMax1/2
  Calculate Point Features/1(F) -> F/1

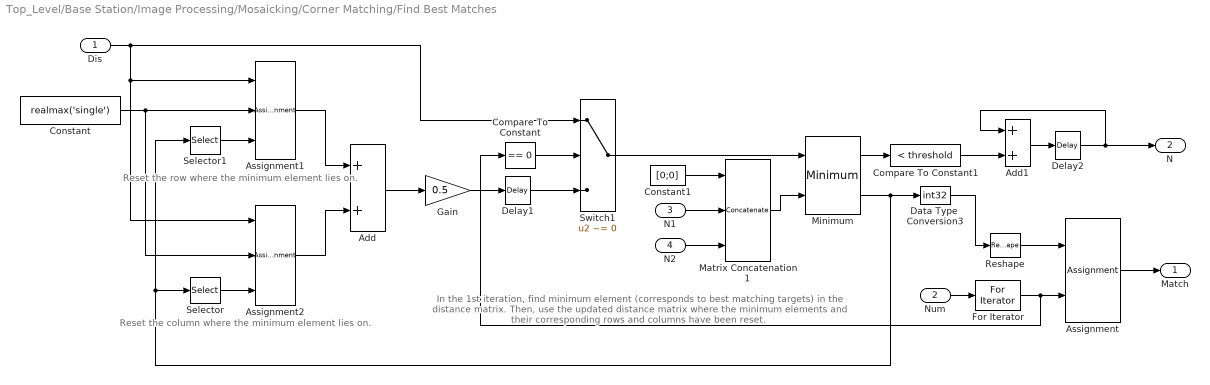
== system Top_Level/Base Station/Image Processing/Mosaicking/Corner Matching/Find Best Matches ==
  note: In the 1st iteration, find minimum element (corresponds to
      | best matching targets) in the distance matrix. Then, use the
      | updated distance matrix where the minimum elements and
      | their  corresponding rows and columns have been reset.
  note: Reset the column where the
      | minimum element lies on.
  note: Reset the row where the
      | minimum element lies on.
  Dis : Inport  OutDataType=sfix(16)  OutScaling=2^0
  Num : Inport  Port=2  OutDataType=sfix(16)  OutScaling=2^0
  N1 : Inport  Port=3  OutDataType=sfix(16)  OutScaling=2^0
  N2 : Inport  Port=4  OutDataType=sfix(16)  OutScaling=2^0
  Add : Sum  OutDataType=sfix(16)  OutScaling=2^-10
  Add1 : Sum  OutDataTypeMode=int32  OutDataType=sfix(16)  OutScaling=2^-10  OutDataTypeStr=int32
  Assignment : Assignment  NumberOfDimensions=2  IndexMode=Zero-based  OutputInitialize=Specify size for each dimension in table  IndexOptions=Assign all,Index vector (port)  Indices=-1,-1  OutputSizes=2,maxNum
  Assignment1 : Assignment  NumberOfDimensions=2  IndexMode=Zero-based  IndexOptions=Index vector (port),Assign all  Indices=1,-1  OutputSizes=1,1
  Assignment2 : Assignment  NumberOfDimensions=2  IndexMode=Zero-based  IndexOptions=Assign all,Index vector (port)  Indices=-1,-1  OutputSizes=1,1
  Compare To Constant : simulink/Logic and Bit Operations/Compare To Constant  SystemSampleTime=-1  relop===  const=0  LogicOutDataTypeMode=boolean  ZeroCross=off
  Compare To Constant1 : simulink/Logic and Bit Operations/Compare To Constant  SystemSampleTime=-1  relop=<  const=threshold  LogicOutDataTypeMode=uint8  ZeroCross=off
  Constant : Constant  Value=realmax('single')  VectorParams1D=off  OutDataType=sfix(16)  OutScaling=2^0  OutDataTypeStr=Inherit: Inherit via back propagation
  Constant1 : Constant  Value=[0;0]  VectorParams1D=off  OutDataType=sfix(16)  OutScaling=2^0  OutDataTypeStr=Inherit: Inherit via back propagation
  Data Type  Conversion3 : DataTypeConversion  OutDataTypeMode=int32  OutDataType=sfix(16)  OutScaling=2^0  OutDataTypeStr=int32  SaturateOnIntegerOverflow=on  RndMeth=Zero
  Delay1 : dspsigops/Delay  dly_unit=Samples  delay=1  ic_detail=off  dif_ic_for_ch=off  dif_ic_for_dly=off  ic=0  reset_popup=None
  Delay2 : dspsigops/Delay  dly_unit=Samples  delay=1  ic_detail=off  dif_ic_for_ch=off  dif_ic_for_dly=off  ic=0  reset_popup=None
  For Iterator : ForIterator  ResetStates=reset  IterationSource=external  IterationLimit=expLaneNum  IndexMode=Zero-based
  Gain : Gain  Gain=0.5  ParameterDataType=sfix(16)  ParameterScaling=2^0  OutDataType=sfix(16)  OutScaling=2^0
  Matrix Concatenation1 : Concatenate  NumInputs=3  Mode=Multidimensional array
  Minimum : dspstat3/Minimum  DialogController=dspDDGCreate  DialogControllerArgs=DataTag7  fcn=Value and Index  reset=None  indexBase=Zero  operateOver=Entire input  Dimension=1  colComp=on  operation=minimum  roiEnable=on  roiType=Rectangles  roiPortion=Entire ROI  roiOutput=Individual statistics for each ROI  roiFlag=off  roundingMode=Floor  overflowMode=off
  Reshape : Reshape  OutputDimensionality=Column vector (2-D)
  Selector : Selector  IndexMode=Zero-based  InputPortWidth=2  IndexOptions=Index vector (dialog)  Indices=1  OutputSizes=1
  Selector1 : Selector  IndexMode=Zero-based  InputPortWidth=2  IndexOptions=Index vector (dialog)  Indices=0  OutputSizes=1
  Switch1 : Switch  Criteria=u2 ~= 0  OutDataType=sfix(16)  OutScaling=2^0
  Match : Outport  OutDataType=sfix(16)  OutScaling=2^0
  N : Outport  Port=2  OutDataType=sfix(16)  OutScaling=2^0
  wires:
  Gain/1 -> Delay1/1
  Minimum/1 -> Compare To Constant1/1
  Compare To Constant1/1 -> Add1/2
  Delay2/1 -> Add1/1, N/1
  Add1/1 -> Delay2/1
  Num/1 -> For Iterator/1
  Data Type  Conversion3/1 -> Reshape/1
  Compare To Constant/1 -> Switch1/2
  For Iterator/1 -> Compare To Constant/1, Assignment/2
  Switch1/1 -> Minimum/1
  Dis/1 -> Switch1/1, Assignment2/1, Assignment1/1
  Delay1/1 -> Switch1/3
  Assignment/1 -> Match/1
  Selector1/1 -> Assignment1/3
  Assignment1/1 -> Add/1
  Assignment2/1 -> Add/2
  Add/1 -> Gain/1
  Minimum/2 -> Data Type  Conversion3/1, Selector/1, Selector1/1
  Constant/1 -> Assignment1/2, Assignment2/2
  Selector/1 -> Assignment2/3
  Constant1/1 -> Matrix Concatenation1/1
  N1/1 -> Matrix Concatenation1/2
  N2/1 -> Matrix Concatenation1/3
  Matrix Concatenation1/1 -> Minimum/2
  Reshape/1 -> Assignment/1

== system Top_Level/Base Station/Image Processing/Mosaicking/Mosaicking/Create ROI ==
  note: Create a rectangle ROI which is the image less its border.
  Image : Inport
  Bias : Bias  Bias=-2
  Matrix Concatenate : Concatenate  Mode=Multidimensional array
  Probe : Probe  ProbeWidth=off  ProbeSampleTime=off  ProbeComplexSignal=off  ProbeSignalDimensions=on  ProbeDimensionsDataType=int32
  Select Height & Width : Selector  IndexMode=Zero-based  InputPortWidth=3  IndexOptions=Index vector (dialog)  Indices=[0 1]  OutputSizes=1
  "[r c]" : Constant  Value=[1 1]  OutDataType=sfix(16)  OutScaling=1  OutDataTypeStr=Inherit: Inherit via back propagation  SampleTime=-1
  ROI : Outport
  wires:
  Probe/1 -> Select Height & Width/1
  Select Height & Width/1 -> Bias/1
  "[r c]"/1 -> Matrix Concatenate/1
  Bias/1 -> Matrix Concatenate/2
  Image/1 -> Probe/1
  Matrix Concatenate/1 -> ROI/1

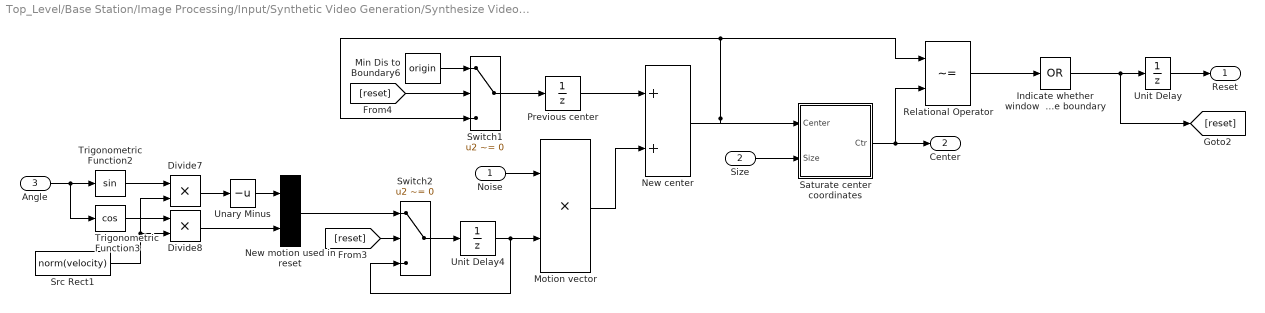
== system Top_Level/Base Station/Image Processing/Input/Synthetic Video Generation/Synthesize Video/Center Locations ==
  Noise : Inport
  Size : Inport  Port=2  OutDataType=sfix(16)  OutScaling=2^0
  Angle : Inport  Port=3
  Divide7 : Product  Inputs=**  OutDataType=sfix(16)  OutScaling=2^-10
  Divide8 : Product  Inputs=**  OutDataType=sfix(16)  OutScaling=2^-10
  Indicate whether window  hit image boundary : Logic  Operator=OR  Inputs=1  AllPortsSameDT=off  OutDataTypeMode=boolean  OutDataTypeStr=boolean
  Min Dis to Boundary6 : Constant  Value=origin  OutDataType=sfix(16)  OutScaling=2^0
  Motion vector : Product  Inputs=**  OutDataType=sfix(16)  OutScaling=2^-10
  New center : Sum  OutDataType=sfix(16)  OutScaling=2^-10
  New motion used in reset : Concatenate  Mode=Vector
  Previous center : UnitDelay  X0=origin  SampleTime=-1
  Relational Operator : RelationalOperator  Operator=~=  LogicOutDataTypeMode=boolean  OutDataTypeStr=boolean
  Saturate center coordinates : Subsystem
  Src Rect1 : Constant  Value=norm(velocity)  VectorParams1D=off  OutDataType=sfix(16)  OutScaling=2^0  OutDataTypeStr=Inherit: Inherit via back propagation
  Switch1 : Switch  Criteria=u2 ~= 0  OutDataType=sfix(16)  OutScaling=2^0
  Switch2 : Switch  Criteria=u2 ~= 0  OutDataType=sfix(16)  OutScaling=2^0
  Trigonometric Function2 : Trigonometry
  Trigonometric Function3 : Trigonometry  Operator=cos
  Unary Minus : UnaryMinus
  Unit Delay : UnitDelay  X0=1  SampleTime=-1
  Unit Delay4 : UnitDelay  X0=velocity  SampleTime=-1
  Reset : Outport
  Center : Outport  Port=2
  wires:
  Unit Delay4/1 -> Switch2/3, Motion vector/2
  Previous center/1 -> New center/1
  [reset] -> Switch1/2
  [reset] -> Switch2/2
  Divide7/1 -> Unary Minus/1
  Unary Minus/1 -> New motion used in reset/1
  Divide8/1 -> New motion used in reset/2
  Src Rect1/1 -> Divide8/2, Divide7/2
  Switch1/1 -> Previous center/1
  Min Dis to Boundary6/1 -> Switch1/1
  Switch2/1 -> Unit Delay4/1
  New motion used in reset/1 -> Switch2/1
  Trigonometric Function3/1 -> Divide8/1
  Trigonometric Function2/1 -> Divide7/1
  Angle/1 -> Trigonometric Function3/1, Trigonometric Function2/1
  Relational Operator/1 -> Indicate whether window  hit image boundary/1
  Indicate whether window  hit image boundary/1 -> [reset], Unit Delay/1
  Saturate center coordinates/1(Ctr) -> Center/1, Relational Operator/2
  Size/1 -> Saturate center coordinates/2(Size)
  New center/1 -> Switch1/3, Relational Operator/1, Saturate center coordinates/1(Center)
  Unit Delay/1 -> Reset/1
  Motion vector/1 -> New center/2
  Noise/1 -> Motion vector/1
